simulink model "ccpitf"  (R2021b)
settings: Solver=VariableStepAuto  StartTime=0.0  StopTime=10.0  RelTol=1e-3
model workspace (MAT data in the model file):
  Ki = 40
  Kp = 800
  b = 50
  m = 1000
  u = 500
settings Model: Creator=feyzi  LastModifiedBy=feyzi

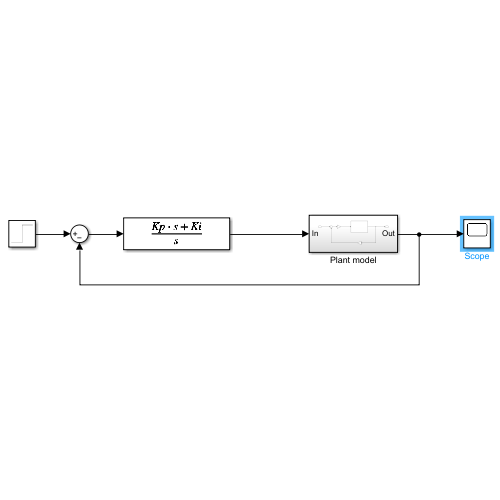
[thumbnail: Simulink's stored preview of the top-level diagram]
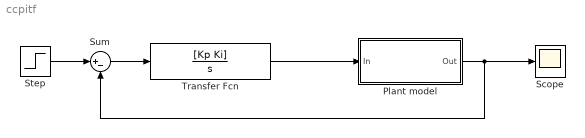
== system ccpitf ==
  Plant model : Subsystem
  Scope : Scope
  Step : Step  Time=0  After=u  SampleTime=0
  Sum : Sum  Inputs=|+-
  Transfer Fcn : TransferFcn  Numerator=[Kp Ki]  Denominator=[1 0]
  wires:
  Plant model/1(Out) -> Scope/1, Sum/2
  Sum/1 -> Transfer Fcn/1
  Transfer Fcn/1 -> Plant model/1(In)
  Step/1 -> Sum/1

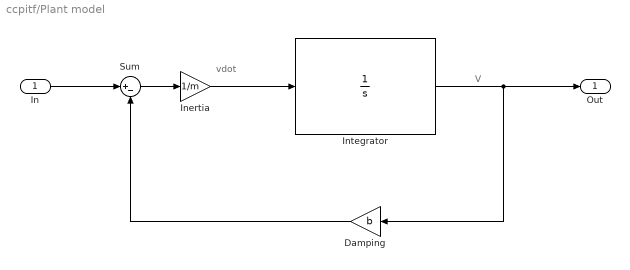
== system ccpitf/Plant model ==
  note: V
  note: vdot
  In : Inport
  Damping : Gain  Gain=b
  Inertia : Gain  Gain=1/m
  Integrator : Integrator  ContinuousStateAttributes="\"Integrator\""
  Sum : Sum  Inputs=|+-
  Out : Outport
  wires:
  Damping/1 -> Sum/2
  Integrator/1 -> Out/1, Damping/1
  In/1 -> Sum/1
  Inertia/1 -> Integrator/1
  Sum/1 -> Inertia/1
